simulink model "ATABEY_sistem_modeli"  (R2025b)
settings: Solver=VariableStepAuto  StartTime=0.0  StopTime=simTime  RelTol=1e-3
undefined symbols (not defined in the file): u1max, u1min, u2max, u2min, u3max, u3min, u4max, u4min, x0
libraries: aerolibfltsims x1, aerolibanimutils x1
settings Model: Creator=erayacikgz  LastModifiedBy=erayacikgz

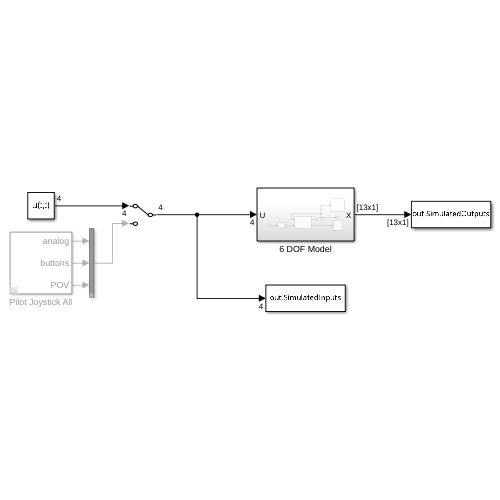
[thumbnail: Simulink's stored preview of the top-level diagram]
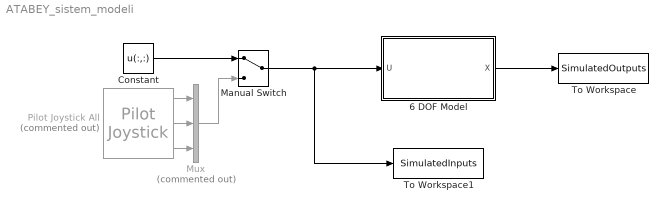
== system ATABEY_sistem_modeli ==
  6 DOF Model : Subsystem
  Constant : Constant  Value=u(:,:)
  Manual Switch : ManualSwitch
  Mux : Mux  Commented=on  Inputs=3
  Pilot Joystick All : aerolibanimutils/Pilot Joystick  Commented=on  JoystickID=Joystick1  OutputConfiguration=AllOutputs  SampleTime=1/30
      settings: LibrarySourceBlock=aerolibanimutils/Pilot Joystick All
  To Workspace : ToWorkspace  VariableName=SimulatedOutputs  SaveFormat=Timeseries  SampleTime=-1
  To Workspace1 : ToWorkspace  VariableName=SimulatedInputs  SaveFormat=Timeseries  SampleTime=-1
  wires:
  6 DOF Model/1(X) -> To Workspace/1
  Manual Switch/1 -> To Workspace1/1, 6 DOF Model/1(U)
  Constant/1 -> Manual Switch/1
  Pilot Joystick All/1 -> Mux/1
  Pilot Joystick All/2 -> Mux/2
  Pilot Joystick All/3 -> Mux/3
  Mux/1 -> Manual Switch/2

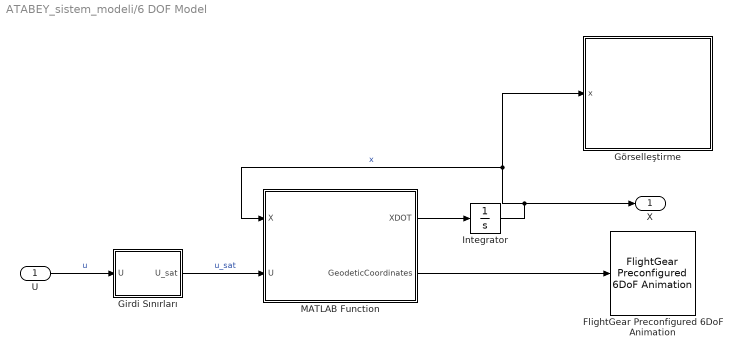
== system ATABEY_sistem_modeli/6 DOF Model ==
  U : Inport
  FlightGear Preconfigured 6DoF Animation : aerolibfltsims/FlightGear Preconfigured 6DoF Animation  xFlightGearVersion=v2019.1  DestinationIpAddress=127.0.0.1  DestinationPort=5502  SampleTime=1/30  packetVersion=24
  Girdi Sınırları : Subsystem
  Görselleştirme : Subsystem
  Integrator : Integrator  InitialCondition=x0(:,:)
  MATLAB Function : MATLAB Function  TreatAsAtomicUnit=on
  X : Outport
  wires:
  MATLAB Function/1(XDOT) -> Integrator/1
  U/1 -> Girdi Sınırları/1(U)  "u"
  Girdi Sınırları/1(U_sat) -> MATLAB Function/2(U)  "u_sat"
  Integrator/1 -> Görselleştirme/1(x), MATLAB Function/1(X), X/1  "x"
  MATLAB Function/2(GeodeticCoordinates) -> FlightGear Preconfigured 6DoF Animation/1

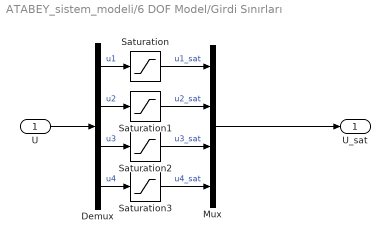
== system ATABEY_sistem_modeli/6 DOF Model/Girdi Sınırları ==
  U : Inport
  Demux : Demux
  Mux : Mux
  Saturation : Saturate  UpperLimit=u1max  LowerLimit=u1min
  Saturation1 : Saturate  UpperLimit=u2max  LowerLimit=u2min
  Saturation2 : Saturate  UpperLimit=u3max  LowerLimit=u3min
  Saturation3 : Saturate  UpperLimit=u4max  LowerLimit=u4min
  U_sat : Outport
  wires:
  Saturation2/1 -> Mux/3  "u3_sat"
  Mux/1 -> U_sat/1
  Demux/2 -> Saturation1/1  "u2"
  Demux/4 -> Saturation3/1  "u4"
  Saturation1/1 -> Mux/2  "u2_sat"
  Saturation/1 -> Mux/1  "u1_sat"
  Saturation3/1 -> Mux/4  "u4_sat"
  Demux/3 -> Saturation2/1  "u3"
  U/1 -> Demux/1
  Demux/1 -> Saturation/1  "u1"

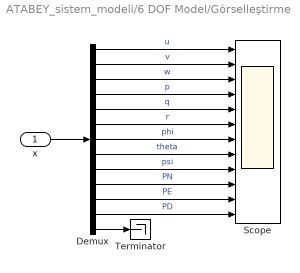
== system ATABEY_sistem_modeli/6 DOF Model/Görselleştirme ==
  x : Inport
  Demux : Demux  Outputs=13
  Scope : Scope  NumInputPorts=12
  Terminator : Terminator
  wires:
  Demux/8 -> Scope/8  "theta"
  Demux/11 -> Scope/11  "PE"
  Demux/3 -> Scope/3  "w"
  Demux/10 -> Scope/10  "PN"
  x/1 -> Demux/1
  Demux/6 -> Scope/6  "r"
  Demux/4 -> Scope/4  "p"
  Demux/7 -> Scope/7  "phi"
  Demux/5 -> Scope/5  "q"
  Demux/1 -> Scope/1  "u"
  Demux/9 -> Scope/9  "psi"
  Demux/13 -> Terminator/1
  Demux/2 -> Scope/2  "v"
  Demux/12 -> Scope/12  "PD"

== matlab function ATABEY_sistem_modeli/6 DOF Model/MATLAB Function ==
  data: X input double size=[13 1]; XDOT output double size=[13 1]; U input double size=[4 1]; GeodeticCoordinates output
function [XDOT, GeodeticCoordinates] = ATABEY_model(X, U)

    [XDOT, GeodeticCoordinates] = ATABEY_dynamics(X, U);
    
end
